simulink model "new_lpp_sim_matfile"  (R2020b)
settings: Solver=FixedStepAuto  StartTime=0.0  StopTime=10  RelTol=1e-3
model workspace (MAT data in the model file):
  firstWarning = 0
  originalScenarioChecksum = 'BB26149F04DD212FFA2CE6E92433E31F'
values from neighbouring files (symbols this model uses):
  lr = 1.6    [localpathplanning_DDPG2.m]
  m = 1575    [localpathplanning_DDPG2.m]
libraries: drivingscenarioandsensors x6, sim3dautolib x3, rllib x1, sim3dlib x1, autolibshared x1
settings Model: Creator=ubuntu  LastModifiedBy=leh

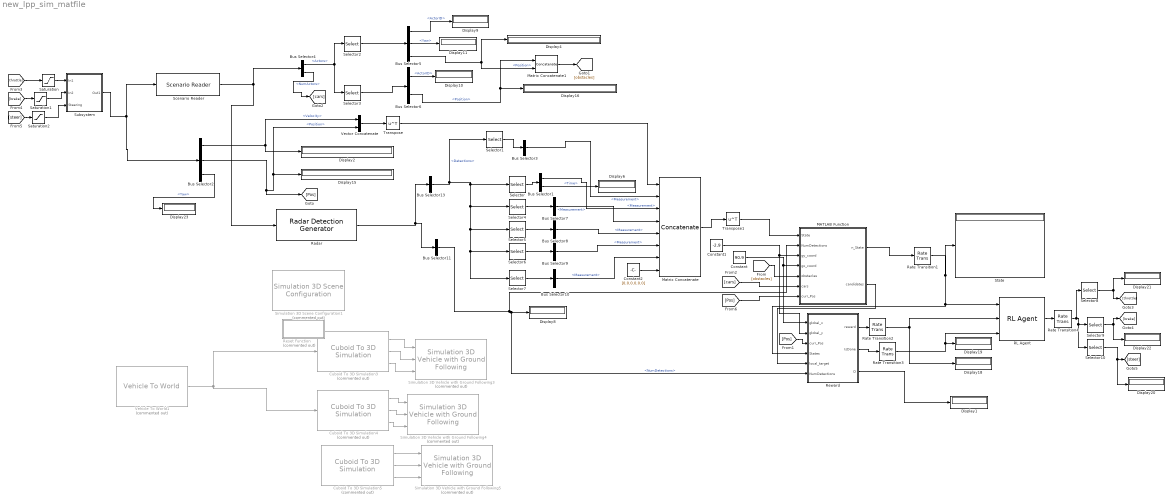
== system new_lpp_sim_matfile ==
  Bus Selector1 : BusSelector  OutputSignals=Measurement,Time
  Bus Selector{3,7..10} (5 alike) : BusSelector  OutputSignals=Measurement
  Bus Selector11 : BusSelector  OutputSignals=NumDetections
  Bus Selector13 : BusSelector  OutputSignals=Detections
  Bus Selector2 : BusSelector  OutputSignals=Velocity,Position,Yaw
  Bus Selector4 : BusSelector  OutputSignals=Actors,NumActors
  Bus Selector5 : BusSelector  OutputSignals=ActorID,Yaw,Position
  Bus Selector6 : BusSelector  OutputSignals=ActorID,Position
  Constant : Constant  Value=90.9
  Constant1 : Constant  Value=-2.9
  Constant2 : Constant  Value=[0,0,0,0,0,0]
  Cuboid To 3D Simulation3 : drivingscenarioandsensors/Cuboid To 3D Simulation  Commented=on  SpecifyActorID=on  ActorIDToConvert=2  SimulateUsing=Interpreted execution
      settings: SourceProductBaseCode=DR
  Cuboid To 3D Simulation4 : drivingscenarioandsensors/Cuboid To 3D Simulation  Commented=on  SpecifyActorID=on  ActorIDToConvert=3  SimulateUsing=Interpreted execution
      settings: SourceProductBaseCode=DR
  Cuboid To 3D Simulation5 : drivingscenarioandsensors/Cuboid To 3D Simulation  Commented=on  SpecifyActorID=on  ActorIDToConvert=1  SimulateUsing=Interpreted execution
      settings: SourceProductBaseCode=DR
  Display{1..2,4,6,8..11,15..16,18..23} (16 alike) : Display
  MATLAB Function : MATLAB Function  TreatAsAtomicUnit=on
  Matrix Concatenate : Concatenate  NumInputs=8  Mode=Multidimensional array  ConcatenateDimension=2
  Matrix Concatenate1 : Concatenate  Mode=Multidimensional array
  RL Agent : rllib/RL Agent  Agent=agent  ProvideReward=on  ProvideIsDone=on  ProvideCumRwd=off  TreatAsDirectFeedthrough=on  CollectLoggedSignals=on  CollectModelStates=on
  Radar : drivingscenarioandsensors/Radar Detection Generator  SensorIndex=1  UpdateInterval=0.1  SensorLocation=[3.7 0]  Height=0.2  Yaw=0  Pitch=0  Roll=0  BusNameSource=Auto  BusName=BusRadarDetectionGenerator  MaxNumDetectionsSource=Property  MaxNumDetections=6  DetectionCoordinates=Ego Cartesian  SimulateUsing=Interpreted execution  AzimuthResolution=4  ElevationResolution=10  RangeResolution=2.5  RangeRateResolution=0.5  AzimuthBiasFraction=0.1  ElevationBiasFraction=0.1  RangeBiasFraction=0.05  RangeRateBiasFraction=0.05  FieldOfView=[20 5]  MaxRange=100  RangeRateLimits=[-100 100]  DetectionProbability=0.9  FalseAlarmRate=1e-06  ReferenceRange=50  ReferenceRCS=0  HasElevation=off  HasRangeRate=on  HasNoise=off  HasFalseAlarms=off  HasOcclusion=off  InitialSeedSource=Repeatable  InitialSeed=0  UsedSeed=0  ActorProfilesSource=MATLAB expression  ActorProfilesParameters=driving.internal.ActorProfilesRadarParameters  ActorProfilesExpression=[struct('ActorID',1,'ClassID',1,'Length',4.7,'Width',1.8,'Height',1.4,'OriginOffset',[-1.35 0 0],'MeshVertices',[3.7 -0.9 1.4;3.7 0.9 1.4;-1 0.9 1.4;-1 -0.9 1.4;3.7 -0.9 0;3.7 0.9 0;-1 0.9 0;-1 -0.9 0],'MeshFaces',[6 2 1;1 5 6;8 4 3;3 7 8;6 7 3;3 2 6;5 1 4;4 8 5;4 1 2;2 3 4;7 6 5;5 8 7],'RCSPattern',[10 10;10 10],'RCSAzimuthAngles',[-180 180],'RCSElevationAngles',[-90 90]); struct('ActorID',2,'ClassID',1,'Length',4.7,'Width',1.8,'Height',1.4,'OriginOffset',[-1.35 0 0],'MeshVertices',[3.7 -0.9 1.4;3.7 0.9 1.4;-1 0.9 1.4;-1 -0.9 1.4;3.7 -0.9 0;3.7 0.9 0;-1 0.9 0;-1 -0.9 0],'MeshFaces',[6 2 1;1 5 6;8 4 3;3 7 8;6 7 3;3 2 6;5 1 4;4 8 5;4 1 2;2 3 4;7 6 5;5 8 7],'RCSPattern',[10 10;10 10],'RCSAzimuthAngles',[-180 180],'RCSElevationAngles',[-90 90]); struct('ActorID',3,'ClassID',1,'Length',4.7,'Width',1.8,'Height',1.4,'OriginOffset',[-1.35 0 0],'MeshVertices',[3.7 -0.9 1.4;3.7 0.9 1.4;-1 0.9 1.4;-1 -0.9 1.4;3.7 -0.9 0;3.7 0.9 0;-1 0.9 0;-1 -0.9 0],'MeshFaces',[6 2 1;1 5 6;8 4 3;3 7 8;6 7 3;3 2 6;5 1 4;4 8 5;4 1 2;2 3 4;7 6 5;5 8 7],'RCSPattern',[10 10;10 10],'RCSAzimuthAngles',[-180 180],'RCSElevationAngles',[-90 90])]
      settings: SourceProductBaseCode=DR
  Rate Transition{1..4} (4 alike) : RateTransition
  Reset Function : Subsystem  Commented=on  TreatAsAtomicUnit=on
  Reward : Subsystem
  Saturation : Saturate  UpperLimit=10  LowerLimit=0
  Saturation1 : Saturate  UpperLimit=10  LowerLimit=0
  Saturation2 : Saturate  UpperLimit=180  LowerLimit=-180
  Scenario Reader : drivingscenarioandsensors/Scenario Reader  ScenarioSource=From workspace  ScenarioFileName=C:\Users\leh\Desktop\RL_LPP\temp_lpp_env.mat  ScenarioVariableName=scenario1  OutputCoordinateSystem=Vehicle coordinates  EgoVehicleSource=Input port  EgoVehicleActorID=1  OrientVehiclesOnRoad=off  OutputEgoVehiclePose=off  SampleTime=0.1  LaneBoundaryOutput=None  LaneBoundaryDistance=0:0.5:9.5  LaneBoundaryLocation=Center of lane markings  BusNameSource=Auto  BusName=BusActors  BusName2Source=Auto  BusName2=BusLaneBoundaries  BusName3Source=Auto  BusName3=BusEgoActor  ShowCoordinateLabels=on  SimulateUsing=Interpreted execution
  Selector : Selector  NumberOfDimensions=2  InputPortWidth=3  IndexOptions=Index vector (dialog),Index vector (dialog)  Indices=[1],[1]  OutputSizes=1,1
  Selector1 : Selector  NumberOfDimensions=2  InputPortWidth=3  IndexOptions=Index vector (dialog),Index vector (dialog)  Indices=[2],[1]  OutputSizes=1,1
  Selector10 : Selector  NumberOfDimensions=2  InputPortWidth=3  IndexOptions=Index vector (dialog),Index vector (dialog)  Indices=[3],[1]  OutputSizes=1,1
  Selector2 : Selector  NumberOfDimensions=2  InputPortWidth=3  IndexOptions=Index vector (dialog),Index vector (dialog)  Indices=[2],[1]  OutputSizes=1,1
  Selector3 : Selector  NumberOfDimensions=2  InputPortWidth=3  IndexOptions=Index vector (dialog),Index vector (dialog)  Indices=[1],[1]  OutputSizes=1,1
  Selector4 : Selector  NumberOfDimensions=2  InputPortWidth=3  IndexOptions=Index vector (dialog),Index vector (dialog)  Indices=[3],[1]  OutputSizes=1,1
  Selector5 : Selector  NumberOfDimensions=2  InputPortWidth=3  IndexOptions=Index vector (dialog),Index vector (dialog)  Indices=[4],[1]  OutputSizes=1,1
  Selector6 : Selector  NumberOfDimensions=2  InputPortWidth=3  IndexOptions=Index vector (dialog),Index vector (dialog)  Indices=[5],[1]  OutputSizes=1,1
  Selector7 : Selector  NumberOfDimensions=2  InputPortWidth=3  IndexOptions=Index vector (dialog),Index vector (dialog)  Indices=[6],[1]  OutputSizes=1,1
  Selector8 : Selector  NumberOfDimensions=2  InputPortWidth=3  IndexOptions=Index vector (dialog),Index vector (dialog)  Indices=[1],[1]  OutputSizes=1,1
  Selector9 : Selector  NumberOfDimensions=2  InputPortWidth=3  IndexOptions=Index vector (dialog),Index vector (dialog)  Indices=[2],[1]  OutputSizes=1,1
  Simulation 3D Scene Configuration1 : sim3dlib/Simulation 3D Scene Configuration  Priority=0  Commented=on  ProjectFormat=Default Scenes  SceneDesc=Straight road  ProjectName=VehicleSimulation.exe  ScenePath=/Game/Maps/HwStrght  vehTagList={'Car';'Car1';'Car2';'Scene Origin'}  vehTag=Car  OpVisEn=off  Ts=0.1  EnableWindow=on  sensorTag=MainCamera2  sensorId=2  sensorName=MainCamera2  mountLoc=Origin  offsetFlag=off  tmountOffset=[0, 0, 0]  rmountOffset=[0, 0, 0]  HorizontalResolution=1280  VerticalResolution=720  HorizontalFOV=60  mountPoint=[0 0 0]  mountOrientation=[0 0 0]  aMode=3  ID=2
      settings: SourceProductBaseCode=DR,UV,VE
  Simulation 3D Vehicle with Ground Following3 : sim3dautolib/Simulation 3D Vehicle with Ground Following  Priority=-1  Commented=on  PassVehMesh=Sedan  VehColor=Orange  InitialPos=[6.6, 0.4, 0]  InitialRot=[0, 0, 2.51]  ActorName=Car1  SampleTime=0.1  ActorType=SimulinkVehicle  ID=C  aMode=3  ActorTag=Car1  CoordinateScheme=ISO  TransformOutportEnabled=off
      settings: SourceProductBaseCode=DR,UV,VE
  Simulation 3D Vehicle with Ground Following4 : sim3dautolib/Simulation 3D Vehicle with Ground Following  Priority=-1  Commented=on  PassVehMesh=Sedan  VehColor=Yellow  InitialPos=[38.3, -2.5, 0]  InitialRot=[0, 0, 0]  ActorName=Car2  SampleTime=0.1  ActorType=SimulinkVehicle  ID=C  aMode=3  ActorTag=Car2  CoordinateScheme=ISO  TransformOutportEnabled=off
      settings: SourceProductBaseCode=DR,UV,VE
  Simulation 3D Vehicle with Ground Following5 : sim3dautolib/Simulation 3D Vehicle with Ground Following  Priority=-1  Commented=on  PassVehMesh=Sedan  VehColor=Blue  InitialPos=[1.3, -2.7, 0]  InitialRot=[0, 0, 0]  ActorName=Car  SampleTime=0.1  ActorType=SimulinkVehicle  ID=C  aMode=3  ActorTag=Car  CoordinateScheme=ISO  TransformOutportEnabled=off
      settings: SourceProductBaseCode=DR,UV,VE
  State : Display
  Subsystem : Subsystem
  Transpose : Math  Operator=transpose  SaturateOnIntegerOverflow=on
  Transpose1 : Math  Operator=transpose  SaturateOnIntegerOverflow=on
  Vector Concatenate : Concatenate
  Vehicle To World1 : drivingscenarioandsensors/Vehicle To World  Commented=on  BusNameSource=Auto  BusName=BusVehicleToWorldActors  SimulateUsing=Interpreted execution
      settings: SourceProductBaseCode=DR
  wires:
  Bus Selector1/2 -> Display6/1  "<Time>"
  Bus Selector13/1 -> Selector7/1, Selector6/1, Selector5/1, Selector4/1, Selector/1, Selector1/1  "<Detections>"
  Bus Selector1/1 -> Matrix Concatenate/3  "<Measurement>"
  Selector/1 -> Bus Selector1/1
  Selector1/1 -> Bus Selector3/1
  Bus Selector4/1 -> Selector3/1, Selector2/1  "<Actors>"
  Selector2/1 -> Bus Selector5/1
  Bus Selector5/1 -> Display9/1  "<ActorID>"
  Selector3/1 -> Bus Selector6/1
  Bus Selector6/1 -> Display10/1  "<ActorID>"
  Bus Selector5/2 -> Display11/1  "<Yaw>"
  Bus Selector5/3 -> Matrix Concatenate1/2, Display4/1  "<Position>"
  Bus Selector3/1 -> Matrix Concatenate/2  "<Measurement>"
  Selector4/1 -> Bus Selector7/1
  Bus Selector7/1 -> Matrix Concatenate/4  "<Measurement>"
  Selector5/1 -> Bus Selector8/1
  Bus Selector8/1 -> Matrix Concatenate/5  "<Measurement>"
  Selector6/1 -> Bus Selector9/1
  Bus Selector9/1 -> Matrix Concatenate/6  "<Measurement>"
  Selector7/1 -> Bus Selector10/1
  Bus Selector10/1 -> Matrix Concatenate/7  "<Measurement>"
  Bus Selector2/2 -> [Pos], Vector Concatenate/2, Display15/1  "<Position>"
  Vector Concatenate/1 -> Transpose/1
  Transpose/1 -> Matrix Concatenate/1
  Matrix Concatenate/1 -> Transpose1/1
  Transpose1/1 -> MATLAB Function/1(State)
  Bus Selector4/2 -> [cars]  "<NumActors>"
  [cars] -> MATLAB Function/6(cars)
  Bus Selector6/2 -> Matrix Concatenate1/1, Display16/1  "<Position>"
  [obstacles] -> MATLAB Function/5(obstacles)
  Matrix Concatenate1/1 -> [obstacles]
  MATLAB Function/2(candidates) -> Reward/5(local_target)
  Constant2/1 -> Matrix Concatenate/8
  MATLAB Function/1(n_State) -> Rate Transition1/1
  Constant/1 -> Reward/1(global_x), MATLAB Function/4(gx_coord)
  Constant1/1 -> Reward/2(global_y), MATLAB Function/3(gy_coord)
  [Pos] -> Reward/3(curr_Pos)
  Reward/1(reward) -> Rate Transition2/1
  Reward/2(IsDone) -> Rate Transition3/1
  Bus Selector2/1 -> Display2/1, Vector Concatenate/1  "<Velocity>"
  Bus Selector2/3 -> Display23/1  "<Yaw>"
  [steer] -> Saturation2/1
  [Pos] -> MATLAB Function/7(curr_Pos)
  Cuboid To 3D Simulation5/1 -> Simulation 3D Vehicle with Ground Following5/1
  Cuboid To 3D Simulation5/3 -> Simulation 3D Vehicle with Ground Following5/3
  Cuboid To 3D Simulation5/2 -> Simulation 3D Vehicle with Ground Following5/2
  Cuboid To 3D Simulation3/3 -> Simulation 3D Vehicle with Ground Following3/3
  Subsystem/1(Out1) -> Scenario Reader/1, Bus Selector2/1
  Cuboid To 3D Simulation4/2 -> Simulation 3D Vehicle with Ground Following4/2
  Cuboid To 3D Simulation4/3 -> Simulation 3D Vehicle with Ground Following4/3
  Cuboid To 3D Simulation4/1 -> Simulation 3D Vehicle with Ground Following4/1
  Cuboid To 3D Simulation3/2 -> Simulation 3D Vehicle with Ground Following3/2
  Vehicle To World1/1 -> Cuboid To 3D Simulation3/1, Cuboid To 3D Simulation4/1
  Cuboid To 3D Simulation3/1 -> Simulation 3D Vehicle with Ground Following3/1
  Selector8/1 -> [throttle], Display21/1
  Selector9/1 -> [brake], Display22/1
  Selector10/1 -> Display20/1, [steer]
  Bus Selector11/1 -> MATLAB Function/2(NumDetections), Reward/6(NumDetections), Display8/1  "<NumDetections>"
  [brake] -> Saturation1/1
  [throttle] -> Saturation/1
  Radar/1 -> Bus Selector11/1, Bus Selector13/1
  Scenario Reader/1 -> Bus Selector4/1, Radar/1
  Rate Transition1/1 -> Reward/4(States), RL Agent/1, State/1
  Rate Transition2/1 -> Display18/1, RL Agent/2
  Rate Transition3/1 -> RL Agent/3, Display19/1
  RL Agent/1 -> Rate Transition4/1
  Saturation/1 -> Subsystem/1(In1)
  Saturation1/1 -> Subsystem/2(In2)
  Saturation2/1 -> Subsystem/3(Steering)
  Rate Transition4/1 -> Selector8/1, Selector10/1, Selector9/1
  Reward/3(D) -> Display1/1

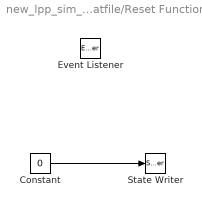
== system new_lpp_sim_matfile/Reset Function ==
  Constant : Constant  Value=0
  Event Listener : EventListener  DisableCoverage=on  EventType=Reset  EventName=reset
  State Writer : StateWriter
  wires:
  Constant/1 -> State Writer/1

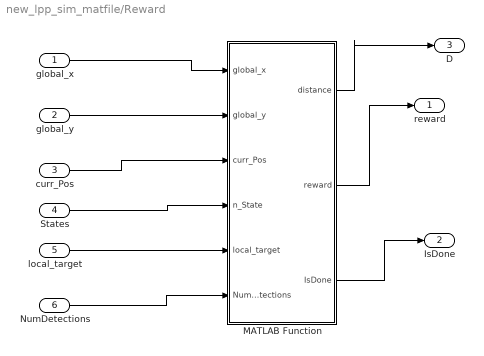
== system new_lpp_sim_matfile/Reward ==
  global_x : Inport
  global_y : Inport  Port=2
  curr_Pos : Inport  Port=3
  States : Inport  Port=4
  local_target : Inport  Port=5
  NumDetections : Inport  Port=6
  MATLAB Function : MATLAB Function  TreatAsAtomicUnit=on
  reward : Outport
  IsDone : Outport  Port=2
  D : Outport  Port=3
  wires:
  global_x/1 -> MATLAB Function/1(global_x)
  global_y/1 -> MATLAB Function/2(global_y)
  curr_Pos/1 -> MATLAB Function/3(curr_Pos)
  States/1 -> MATLAB Function/4(n_State)
  local_target/1 -> MATLAB Function/5(local_target)
  MATLAB Function/3(IsDone) -> IsDone/1
  MATLAB Function/2(reward) -> reward/1
  MATLAB Function/1(distance) -> D/1
  NumDetections/1 -> MATLAB Function/6(NumDetections)

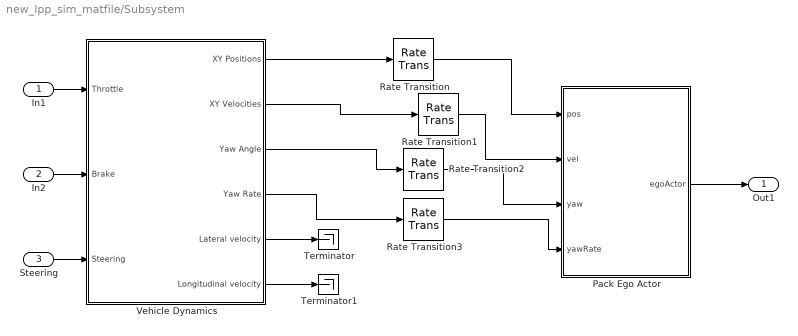
== system new_lpp_sim_matfile/Subsystem ==
  In1 : Inport
  In2 : Inport  Port=2
  Steering : Inport  Port=3
  Pack Ego Actor : MATLAB Function  TreatAsAtomicUnit=on
  Rate Transition{,1..3} (4 alike) : RateTransition
  Terminator : Terminator
  Terminator1 : Terminator
  Vehicle Dynamics : Subsystem  VariantControl=Variant2
  Out1 : Outport
  wires:
  Vehicle Dynamics/4(Yaw Rate) -> Rate Transition3/1
  Rate Transition/1 -> Pack Ego Actor/1(pos)
  Vehicle Dynamics/2(XY Velocities) -> Rate Transition1/1
  Vehicle Dynamics/1(XY Positions) -> Rate Transition/1
  Rate Transition1/1 -> Pack Ego Actor/2(vel)
  Pack Ego Actor/1(egoActor) -> Out1/1
  Rate Transition3/1 -> Pack Ego Actor/4(yawRate)
  Vehicle Dynamics/3(Yaw Angle) -> Rate Transition2/1
  In1/1 -> Vehicle Dynamics/1(Throttle)
  In2/1 -> Vehicle Dynamics/2(Brake)
  Rate Transition2/1 -> Pack Ego Actor/3(yaw)
  Vehicle Dynamics/5(Lateral velocity) -> Terminator/1
  Vehicle Dynamics/6(Longitudinal velocity) -> Terminator1/1
  Steering/1 -> Vehicle Dynamics/3(Steering)

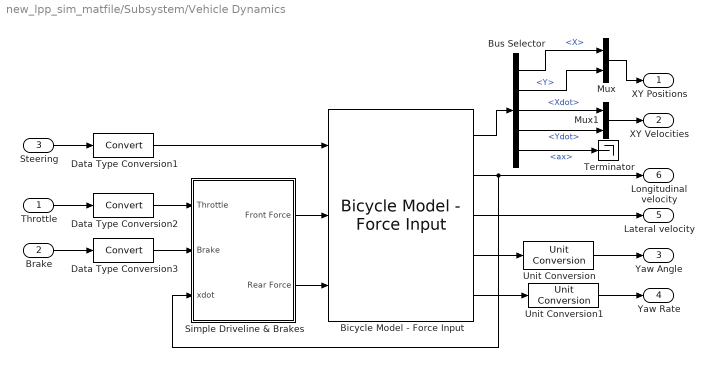
== system new_lpp_sim_matfile/Subsystem/Vehicle Dynamics ==
  Throttle : Inport  Unit=m/s^2
  Brake : Inport  Port=2  Unit=m/s^2
  Steering : Inport  Port=3  Unit=rad
  Bicycle Model - Force Input : autolibshared/Bicycle Model - Force Input  trackMode=Single (bicycle)  inputMode=External longitudinal forces  frontSteerMode=on  rearSteerMode=off  windMode=off  muMode=off  extFMode=off  extMMode=off  aMode=3  NF=2  NR=2  m=m  a=lf  b=lr  h=0.35  X_o=ego_x  xdot_o=ego_v  CalphaMode=off  sigmaMode=on  w=[1.4,1.4]  Cy_f=19000  Cy_r=33000  sigma_f=.1  sigma_r=.1  alpha_f_brk=[-.1 .1]  Cy_f_data=[-9e3 9e3]  alpha_r_brk=[-.1 .1]  Cy_r_data=[-9e3 9e3]  Y_o=ego_y  ydot_o=0  Izz=lz  psi_o=ego_yaw  r_o=0  Af=0  Cd=.3  Cl=.1  Cpm=.1  beta_w=[0:0.01:0.3]  Cs=[0:0.03:0.9]  Cym=[0:0.01:0.3]  Pabs=101325  Tair=273  g=9.81  mu=1  xdot_tol=.01  Fznom=5000  Fxtire_sat=1e6  Fytire_sat=1e6  longOff=0  latOff=0  vertOff=0
      settings: SourceProductBaseCode=PW,MT,UV,VE,VP
  Bus Selector : BusSelector  OutputSignals=InertFrm.FrntAxl.Disp.X,InertFrm.FrntAxl.Disp.Y,InertFrm.FrntAxl.Vel.Xdot,InertFrm.FrntAxl.Vel.Ydot,BdyFrm.Cg.Acc.ax
  Data Type Conversion1 : DataTypeConversion
  Data Type Conversion2 : DataTypeConversion
  Data Type Conversion3 : DataTypeConversion
  Mux : Mux  Inputs=2
  Mux1 : Mux  Inputs=2
  Simple Driveline & Brakes : Subsystem
  Terminator : Terminator
  Unit Conversion : UnitConversion  OutputType=Inherit: Inherit via back propagation
  Unit Conversion1 : UnitConversion  OutputType=Inherit: Inherit via back propagation
  XY Positions : Outport  Unit=m  VectorParamsAs1DForOutWhenUnconnected=off
  XY Velocities : Outport  Port=2  Unit=m/s  VectorParamsAs1DForOutWhenUnconnected=off
  Yaw Angle : Outport  Port=3  Unit=deg  VectorParamsAs1DForOutWhenUnconnected=off
  Yaw Rate : Outport  Port=4  Unit=degree/s  VectorParamsAs1DForOutWhenUnconnected=off
  Lateral velocity : Outport  Port=5  VectorParamsAs1DForOutWhenUnconnected=off
  Longitudinal velocity : Outport  Port=6  VectorParamsAs1DForOutWhenUnconnected=off
  wires:
  Unit Conversion1/1 -> Yaw Rate/1
  Mux1/1 -> XY Velocities/1
  Mux/1 -> XY Positions/1
  Bicycle Model - Force Input/1 -> Bus Selector/1
  Bus Selector/3 -> Mux1/1  "<Xdot>"
  Bicycle Model - Force Input/2 -> Longitudinal velocity/1, Simple Driveline & Brakes/3(xdot)
  Bus Selector/2 -> Mux/2  "<Y>"
  Bicycle Model - Force Input/4 -> Unit Conversion/1
  Bus Selector/4 -> Mux1/2  "<Ydot>"
  Bicycle Model - Force Input/5 -> Unit Conversion1/1
  Unit Conversion/1 -> Yaw Angle/1
  Bus Selector/1 -> Mux/1  "<X>"
  Steering/1 -> Data Type Conversion1/1
  Throttle/1 -> Data Type Conversion2/1
  Data Type Conversion1/1 -> Bicycle Model - Force Input/1
  Simple Driveline & Brakes/1(Front Force) -> Bicycle Model - Force Input/2
  Simple Driveline & Brakes/2(Rear Force) -> Bicycle Model - Force Input/3
  Bicycle Model - Force Input/3 -> Lateral velocity/1
  Data Type Conversion2/1 -> Simple Driveline & Brakes/1(Throttle)
  Brake/1 -> Data Type Conversion3/1
  Data Type Conversion3/1 -> Simple Driveline & Brakes/2(Brake)
  Bus Selector/5 -> Terminator/1  "<ax>"

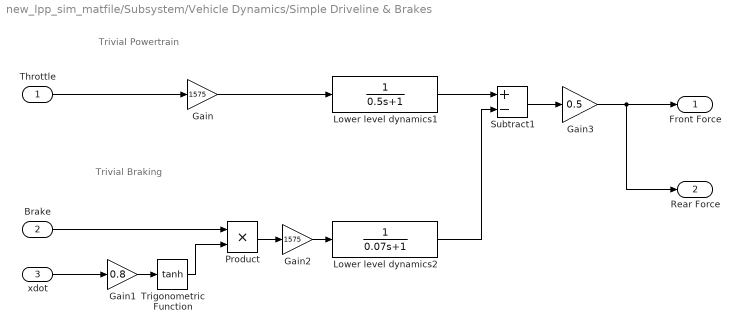
== system new_lpp_sim_matfile/Subsystem/Vehicle Dynamics/Simple Driveline & Brakes ==
  note: Trivial Powertrain
  note: Trivial Braking
  Throttle : Inport
  Brake : Inport  Port=2
  xdot : Inport  Port=3
  Gain : Gain  Gain=1575
  Gain1 : Gain  Gain=0.8
  Gain2 : Gain  Gain=1575
  Gain3 : Gain  Gain=0.5
  Lower level dynamics1 : TransferFcn  Denominator=[0.5 1]
  Lower level dynamics2 : TransferFcn  Denominator=[0.07 1]
  Product : Product
  Subtract1 : Sum  Inputs=+-
  Trigonometric Function : Trigonometry  Operator=tanh
  Front Force : Outport  VectorParamsAs1DForOutWhenUnconnected=off
  Rear Force : Outport  Port=2  VectorParamsAs1DForOutWhenUnconnected=off
  wires:
  Gain3/1 -> Rear Force/1, Front Force/1
  Brake/1 -> Product/1
  Throttle/1 -> Gain/1
  Gain2/1 -> Lower level dynamics2/1
  Gain/1 -> Lower level dynamics1/1
  Subtract1/1 -> Gain3/1
  xdot/1 -> Gain1/1
  Product/1 -> Gain2/1
  Trigonometric Function/1 -> Product/2
  Gain1/1 -> Trigonometric Function/1
  Lower level dynamics1/1 -> Subtract1/1
  Lower level dynamics2/1 -> Subtract1/2

== matlab function new_lpp_sim_matfile/Reward/MATLAB Function ==
  data: distance output; global_x input; reward output; global_y input; curr_Pos input; n_State input; local_target input; IsDone output; NumDetections input
function [distance,reward, IsDone] = Reward(global_x,global_y,curr_Pos,n_State,local_target,NumDetections)
distance = 0;
rad_Pos = n_State(3:8,1:2); % relative coordinates of obstacles detected in radar. The radar is the origin
IsDone = 0;
%curr_Pos_y1 = curr_Pos(1,2) + 1.6;
%curr_Pos_y2 = curr_Pos(1,2) - 1.6;
curr_Pos (1,1);
%% claculate reward

if curr_Pos(1,2) >= 2 || curr_Pos(1,2) <= -4.075 % if current position of ego car cross over the line of lane this episode is done.
    
    reward = -10;
    IsDone = 1;
    
    
else
    reward = 1;
    current_x = (global_x - curr_Pos(1,1)).^2; % if distance between global and current position less than 1m reward is 20.
    current_y = (global_y - curr_Pos(1,2)).^2;
    current_d = sqrt(current_x + current_y);
    
    local_x = (global_x - local_target(1,1)).^2; % if distance between local and global position less than 1m reward is 10.
    local_y = (global_y - local_target(1,2)).^2;
    local_d = sqrt(local_x + local_y);
    
    if current_d <= 1
        reward = reward + 50;
        IsDone = 1;
    

    elseif local_d <= 1
            reward = (-0.01 * (current_d)) + reward; % if current_d = 80m this step get +0.2 reward score
            IsDone = 0;
        
    elseif current_d > 1 && local_d > 1 && NumDetections ~= 0
        for i = 1:length(rad_Pos)
            if rad_Pos(i,1) == 0 && rad_Pos(i,2) == 0 % Nothing detected
                reward = 0;
                IsDone = 0;
                %continue
            else
                d_x = (rad_Pos(i,1))^2 ;
                d_y = (rad_Pos(i,2))^2 ;
                distance = sqrt(d_x + d_y);
                
                if distance > 3.7
                    reward = (-0.01 * (current_d + reward)); % if current_d = 80m this step get -0.81 reward score
                    IsDone = 0;
                
                elseif distance <= 3.7
                    reward = -(reward - distance);
                    IsDone = 1;
                end
            end
        end
    elseif current_d > 1 && local_d > 1 && NumDetections == 0
        reward = (-0.01 * (current_d)) + reward;
    end
end

== matlab function new_lpp_sim_matfile/MATLAB Function ==
  data: n_State output; State input; NumDetections input; gy_coord input; gx_coord input; obstacles input; cars input; candidates output; curr_Pos input
function [n_State, candidates] = createState(State,NumDetections,gy_coord,gx_coord,obstacles,cars,curr_Pos)

%size = length(temp_State(2:6,:));
%curr_pos = temp_State(1,4:5); % ego car's current position
n_State = zeros(9,3);
candidates = zeros(1,2);


current_x = (gx_coord - curr_Pos(1,1)).^2;
current_y = (gy_coord - curr_Pos(1,2)).^2;
current_d = sqrt(current_x + current_y);

% It only works when an obastacle vehicle is caught on the radar sensor.
% This code calculates local target using the global coordinates of the obstacle vehicle
% and the current position of the ego vehicle.
if curr_Pos(1,2) < 2 && curr_Pos(1,2) > -4.075
    if NumDetections ~= 0
    
        for i = 1:cars
            
                
             %   break
        
            if i < cars
                med_x = abs((obstacles(i,1) + obstacles(i+1,1))/2); % middle 
                med_y = abs((obstacles(i,2) + obstacles(i+1,2))/2);
            
                if obstacles(i,1) > obstacles(i+1,1)
                    x_coord = obstacles(i+1,1) + med_x;
                else
                    x_coord = obstacles(i,1) + med_x;
                end
        
                if obstacles(i,2) > obstacles(i+1,2)
                    y_coord = obstacles(i+1,2) + med_y;
                else
                    y_coord = obstacles(i,2) + med_y;
                end
        
                if candidates == 0
                    candidates(1,1) = x_coord;
                    candidates(1,2) = y_coord;
                elseif candidates ~= 0
                    d_1 = sqrt((candidates(1,1) - gx_coord).^2 + (candidates(1,2) - gy_coord).^2);
                    d_2 = sqrt((x_coord -gx_coord).^2 + (y_coord - gy_coord).^2); % distance between global and candidates
                    if abs(d_1) > abs(d_2)
                        candidates(1,1) = x_coord;
                        candidates(1,2) = y_coord;
                    end
                end
            end
        end
    
    %local_target = candidates;
    
    else
        candidates(1,1) = gx_coord;
        candidates(1,2) = gy_coord;
    end
else
    State(8,1:2) = 0;
    
end
n_State(1,1:3) = State(1,1:3);
n_State(2,1:3) = State(1,4:6);
n_State(3:8,:) = State(2:7,1:3);
n_State(9,1:2) = candidates;
n_State(9,3) = current_d;
%State(8,1:2) = candidates;  % candidates is a local target.
%State(8,4) = current_d;
end

== matlab function new_lpp_sim_matfile/Subsystem/Pack Ego Actor ==
  data: pos input; egoActor output Bus: BusActors1Actors size=1; vel input; yaw input; yawRate input
function egoActor = packEgo(pos,vel,yaw,yawRate)
% Pack ego information into a single ego actor bus
%
% Imoprtant note:
% Output is a bus of type BusActors1Actors!!!!! This is the same bus used by the
% Scenario Reader to output an individual actor. If you change the
% output bus name of Scenario Reader, change the output bus name here
% as well by clicking on 'Edit Data' in the menu above.

egoActor = struct(...
    'ActorID',1,...
    'Position', [pos(1) pos(2) 0], ...
    'Velocity', [vel(1) vel(2) 0], ...
    'Roll', 0, ...
    'Pitch', 0, ...
    'Yaw', yaw, ...
    'AngularVelocity', [0 0 yawRate]);
